simulink model "iot_casestudy_1_16"  (R2023a)
settings: Solver=VariableStepAuto  StartTime=0.0  StopTime=3.0  RelTol=1e-3
undefined symbols (not defined in the file or in its folder): m, n
(part 1 of 2)
settings Model: PacingRate=0.089000  Creator=simon  LastModifiedBy=simon
settings DataIOCC: SignalLogging=off
settings OptimizationCC: AccelVerboseBuild=on

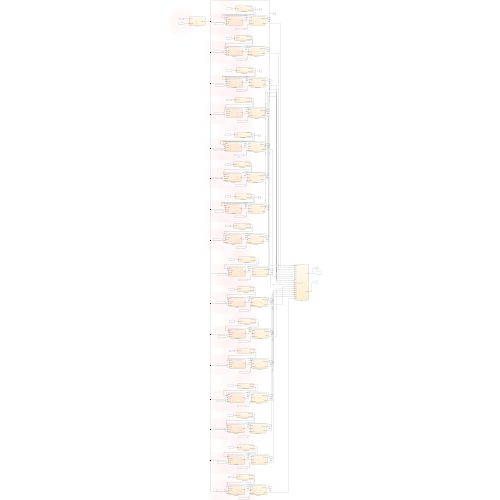
[thumbnail: Simulink's stored preview of the top-level diagram]
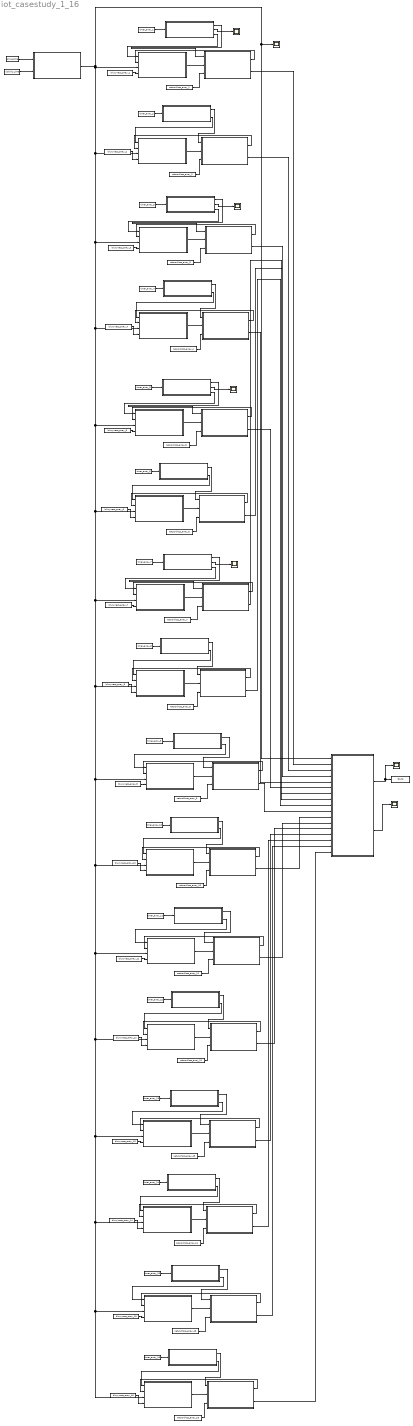
== system iot_casestudy_1_16 ==
  CameraControl : Stateflow chart  TreatAsAtomicUnit=on
      settings: PortSchema="{\"entries\":[{\"content\":{\"sides\":[{\"content\":{\"connectorIds\":[\"In3\",\"In1\",\"In2\"]},\"type\":\"ConnectorPlacement.EquallySpacedRectSide\",\"uuid\":\"ab620818-a51b-4a3c-9b00-600c4a6c30a0\"},{\"content\":{\"connectorIds\":[\"Out1\",\"Out2\"],\"side\":\"RIGHT\"},\"type\":\"ConnectorPlacement.EquallySpacedRectSide\",\"uuid\":\"fd7d4612-1aa1-44dc-acf4-0ffdcf3f06ab\"},{\"content\":{\"side\":\"TOP\"},\"type\":\"ConnectorPlacement.EquallySpacedRectSide\",\"uuid\":\"b173ad78-f658-4e97-9d6b-ed1d410de5f1\"}]},\"type\":\"ConnectorPlacement.EquallySpacedConnector\",\"uuid\":\"5700aeec-8725-4d1d-b13d-0f47828af58c\"}],\"packageUris\":[\"http://schema.mathworks.com/mf0/Connector/R2020b\"],\"version\":\"1.0\"}"
  CameraControl1 : Stateflow chart  TreatAsAtomicUnit=on
      settings: PortSchema="{\"entries\":[{\"content\":{\"sides\":[{\"content\":{\"connectorIds\":[\"In3\",\"In1\",\"In2\"]},\"type\":\"ConnectorPlacement.EquallySpacedRectSide\",\"uuid\":\"ab620818-a51b-4a3c-9b00-600c4a6c30a0\"},{\"content\":{\"connectorIds\":[\"Out1\",\"Out2\"],\"side\":\"RIGHT\"},\"type\":\"ConnectorPlacement.EquallySpacedRectSide\",\"uuid\":\"fd7d4612-1aa1-44dc-acf4-0ffdcf3f06ab\"},{\"content\":{\"side\":\"TOP\"},\"type\":\"ConnectorPlacement.EquallySpacedRectSide\",\"uuid\":\"b173ad78-f658-4e97-9d6b-ed1d410de5f1\"}]},\"type\":\"ConnectorPlacement.EquallySpacedConnector\",\"uuid\":\"5700aeec-8725-4d1d-b13d-0f47828af58c\"}],\"packageUris\":[\"http://schema.mathworks.com/mf0/Connector/R2020b\"],\"version\":\"1.0\"}"
  CameraControl10 : Stateflow chart  TreatAsAtomicUnit=on
      settings: PortSchema="{\"entries\":[{\"content\":{\"sides\":[{\"content\":{\"connectorIds\":[\"In3\",\"In1\",\"In2\"]},\"type\":\"ConnectorPlacement.EquallySpacedRectSide\",\"uuid\":\"ab620818-a51b-4a3c-9b00-600c4a6c30a0\"},{\"content\":{\"connectorIds\":[\"Out1\",\"Out2\"],\"side\":\"RIGHT\"},\"type\":\"ConnectorPlacement.EquallySpacedRectSide\",\"uuid\":\"fd7d4612-1aa1-44dc-acf4-0ffdcf3f06ab\"},{\"content\":{\"side\":\"TOP\"},\"type\":\"ConnectorPlacement.EquallySpacedRectSide\",\"uuid\":\"b173ad78-f658-4e97-9d6b-ed1d410de5f1\"}]},\"type\":\"ConnectorPlacement.EquallySpacedConnector\",\"uuid\":\"5700aeec-8725-4d1d-b13d-0f47828af58c\"}],\"packageUris\":[\"http://schema.mathworks.com/mf0/Connector/R2020b\"],\"version\":\"1.0\"}"
  CameraControl11 : Stateflow chart  TreatAsAtomicUnit=on
      settings: PortSchema="{\"entries\":[{\"content\":{\"sides\":[{\"content\":{\"connectorIds\":[\"In3\",\"In1\",\"In2\"]},\"type\":\"ConnectorPlacement.EquallySpacedRectSide\",\"uuid\":\"ab620818-a51b-4a3c-9b00-600c4a6c30a0\"},{\"content\":{\"connectorIds\":[\"Out1\",\"Out2\"],\"side\":\"RIGHT\"},\"type\":\"ConnectorPlacement.EquallySpacedRectSide\",\"uuid\":\"fd7d4612-1aa1-44dc-acf4-0ffdcf3f06ab\"},{\"content\":{\"side\":\"TOP\"},\"type\":\"ConnectorPlacement.EquallySpacedRectSide\",\"uuid\":\"b173ad78-f658-4e97-9d6b-ed1d410de5f1\"}]},\"type\":\"ConnectorPlacement.EquallySpacedConnector\",\"uuid\":\"5700aeec-8725-4d1d-b13d-0f47828af58c\"}],\"packageUris\":[\"http://schema.mathworks.com/mf0/Connector/R2020b\"],\"version\":\"1.0\"}"
  CameraControl12 : Stateflow chart  TreatAsAtomicUnit=on
      settings: PortSchema="{\"entries\":[{\"content\":{\"sides\":[{\"content\":{\"connectorIds\":[\"In3\",\"In1\",\"In2\"]},\"type\":\"ConnectorPlacement.EquallySpacedRectSide\",\"uuid\":\"ab620818-a51b-4a3c-9b00-600c4a6c30a0\"},{\"content\":{\"connectorIds\":[\"Out1\",\"Out2\"],\"side\":\"RIGHT\"},\"type\":\"ConnectorPlacement.EquallySpacedRectSide\",\"uuid\":\"fd7d4612-1aa1-44dc-acf4-0ffdcf3f06ab\"},{\"content\":{\"side\":\"TOP\"},\"type\":\"ConnectorPlacement.EquallySpacedRectSide\",\"uuid\":\"b173ad78-f658-4e97-9d6b-ed1d410de5f1\"}]},\"type\":\"ConnectorPlacement.EquallySpacedConnector\",\"uuid\":\"5700aeec-8725-4d1d-b13d-0f47828af58c\"}],\"packageUris\":[\"http://schema.mathworks.com/mf0/Connector/R2020b\"],\"version\":\"1.0\"}"
  CameraControl13 : Stateflow chart  TreatAsAtomicUnit=on
      settings: PortSchema="{\"entries\":[{\"content\":{\"sides\":[{\"content\":{\"connectorIds\":[\"In3\",\"In1\",\"In2\"]},\"type\":\"ConnectorPlacement.EquallySpacedRectSide\",\"uuid\":\"ab620818-a51b-4a3c-9b00-600c4a6c30a0\"},{\"content\":{\"connectorIds\":[\"Out1\",\"Out2\"],\"side\":\"RIGHT\"},\"type\":\"ConnectorPlacement.EquallySpacedRectSide\",\"uuid\":\"fd7d4612-1aa1-44dc-acf4-0ffdcf3f06ab\"},{\"content\":{\"side\":\"TOP\"},\"type\":\"ConnectorPlacement.EquallySpacedRectSide\",\"uuid\":\"b173ad78-f658-4e97-9d6b-ed1d410de5f1\"}]},\"type\":\"ConnectorPlacement.EquallySpacedConnector\",\"uuid\":\"5700aeec-8725-4d1d-b13d-0f47828af58c\"}],\"packageUris\":[\"http://schema.mathworks.com/mf0/Connector/R2020b\"],\"version\":\"1.0\"}"
  CameraControl14 : Stateflow chart  TreatAsAtomicUnit=on
      settings: PortSchema="{\"entries\":[{\"content\":{\"sides\":[{\"content\":{\"connectorIds\":[\"In3\",\"In1\",\"In2\"]},\"type\":\"ConnectorPlacement.EquallySpacedRectSide\",\"uuid\":\"ab620818-a51b-4a3c-9b00-600c4a6c30a0\"},{\"content\":{\"connectorIds\":[\"Out1\",\"Out2\"],\"side\":\"RIGHT\"},\"type\":\"ConnectorPlacement.EquallySpacedRectSide\",\"uuid\":\"fd7d4612-1aa1-44dc-acf4-0ffdcf3f06ab\"},{\"content\":{\"side\":\"TOP\"},\"type\":\"ConnectorPlacement.EquallySpacedRectSide\",\"uuid\":\"b173ad78-f658-4e97-9d6b-ed1d410de5f1\"}]},\"type\":\"ConnectorPlacement.EquallySpacedConnector\",\"uuid\":\"5700aeec-8725-4d1d-b13d-0f47828af58c\"}],\"packageUris\":[\"http://schema.mathworks.com/mf0/Connector/R2020b\"],\"version\":\"1.0\"}"
  CameraControl15 : Stateflow chart  TreatAsAtomicUnit=on
      settings: PortSchema="{\"entries\":[{\"content\":{\"sides\":[{\"content\":{\"connectorIds\":[\"In3\",\"In1\",\"In2\"]},\"type\":\"ConnectorPlacement.EquallySpacedRectSide\",\"uuid\":\"ab620818-a51b-4a3c-9b00-600c4a6c30a0\"},{\"content\":{\"connectorIds\":[\"Out1\",\"Out2\"],\"side\":\"RIGHT\"},\"type\":\"ConnectorPlacement.EquallySpacedRectSide\",\"uuid\":\"fd7d4612-1aa1-44dc-acf4-0ffdcf3f06ab\"},{\"content\":{\"side\":\"TOP\"},\"type\":\"ConnectorPlacement.EquallySpacedRectSide\",\"uuid\":\"b173ad78-f658-4e97-9d6b-ed1d410de5f1\"}]},\"type\":\"ConnectorPlacement.EquallySpacedConnector\",\"uuid\":\"5700aeec-8725-4d1d-b13d-0f47828af58c\"}],\"packageUris\":[\"http://schema.mathworks.com/mf0/Connector/R2020b\"],\"version\":\"1.0\"}"
  CameraControl2 : Stateflow chart  TreatAsAtomicUnit=on
      settings: PortSchema="{\"entries\":[{\"content\":{\"sides\":[{\"content\":{\"connectorIds\":[\"In3\",\"In1\",\"In2\"]},\"type\":\"ConnectorPlacement.EquallySpacedRectSide\",\"uuid\":\"ab620818-a51b-4a3c-9b00-600c4a6c30a0\"},{\"content\":{\"connectorIds\":[\"Out1\",\"Out2\"],\"side\":\"RIGHT\"},\"type\":\"ConnectorPlacement.EquallySpacedRectSide\",\"uuid\":\"fd7d4612-1aa1-44dc-acf4-0ffdcf3f06ab\"},{\"content\":{\"side\":\"TOP\"},\"type\":\"ConnectorPlacement.EquallySpacedRectSide\",\"uuid\":\"b173ad78-f658-4e97-9d6b-ed1d410de5f1\"}]},\"type\":\"ConnectorPlacement.EquallySpacedConnector\",\"uuid\":\"5700aeec-8725-4d1d-b13d-0f47828af58c\"}],\"packageUris\":[\"http://schema.mathworks.com/mf0/Connector/R2020b\"],\"version\":\"1.0\"}"
  CameraControl3 : Stateflow chart  TreatAsAtomicUnit=on
      settings: PortSchema="{\"entries\":[{\"content\":{\"sides\":[{\"content\":{\"connectorIds\":[\"In3\",\"In1\",\"In2\"]},\"type\":\"ConnectorPlacement.EquallySpacedRectSide\",\"uuid\":\"ab620818-a51b-4a3c-9b00-600c4a6c30a0\"},{\"content\":{\"connectorIds\":[\"Out1\",\"Out2\"],\"side\":\"RIGHT\"},\"type\":\"ConnectorPlacement.EquallySpacedRectSide\",\"uuid\":\"fd7d4612-1aa1-44dc-acf4-0ffdcf3f06ab\"},{\"content\":{\"side\":\"TOP\"},\"type\":\"ConnectorPlacement.EquallySpacedRectSide\",\"uuid\":\"b173ad78-f658-4e97-9d6b-ed1d410de5f1\"}]},\"type\":\"ConnectorPlacement.EquallySpacedConnector\",\"uuid\":\"5700aeec-8725-4d1d-b13d-0f47828af58c\"}],\"packageUris\":[\"http://schema.mathworks.com/mf0/Connector/R2020b\"],\"version\":\"1.0\"}"
  CameraControl4 : Stateflow chart  TreatAsAtomicUnit=on
      settings: PortSchema="{\"entries\":[{\"content\":{\"sides\":[{\"content\":{\"connectorIds\":[\"In3\",\"In1\",\"In2\"]},\"type\":\"ConnectorPlacement.EquallySpacedRectSide\",\"uuid\":\"ab620818-a51b-4a3c-9b00-600c4a6c30a0\"},{\"content\":{\"connectorIds\":[\"Out1\",\"Out2\"],\"side\":\"RIGHT\"},\"type\":\"ConnectorPlacement.EquallySpacedRectSide\",\"uuid\":\"fd7d4612-1aa1-44dc-acf4-0ffdcf3f06ab\"},{\"content\":{\"side\":\"TOP\"},\"type\":\"ConnectorPlacement.EquallySpacedRectSide\",\"uuid\":\"b173ad78-f658-4e97-9d6b-ed1d410de5f1\"}]},\"type\":\"ConnectorPlacement.EquallySpacedConnector\",\"uuid\":\"5700aeec-8725-4d1d-b13d-0f47828af58c\"}],\"packageUris\":[\"http://schema.mathworks.com/mf0/Connector/R2020b\"],\"version\":\"1.0\"}"
  CameraControl5 : Stateflow chart  TreatAsAtomicUnit=on
      settings: PortSchema="{\"entries\":[{\"content\":{\"sides\":[{\"content\":{\"connectorIds\":[\"In3\",\"In1\",\"In2\"]},\"type\":\"ConnectorPlacement.EquallySpacedRectSide\",\"uuid\":\"ab620818-a51b-4a3c-9b00-600c4a6c30a0\"},{\"content\":{\"connectorIds\":[\"Out1\",\"Out2\"],\"side\":\"RIGHT\"},\"type\":\"ConnectorPlacement.EquallySpacedRectSide\",\"uuid\":\"fd7d4612-1aa1-44dc-acf4-0ffdcf3f06ab\"},{\"content\":{\"side\":\"TOP\"},\"type\":\"ConnectorPlacement.EquallySpacedRectSide\",\"uuid\":\"b173ad78-f658-4e97-9d6b-ed1d410de5f1\"}]},\"type\":\"ConnectorPlacement.EquallySpacedConnector\",\"uuid\":\"5700aeec-8725-4d1d-b13d-0f47828af58c\"}],\"packageUris\":[\"http://schema.mathworks.com/mf0/Connector/R2020b\"],\"version\":\"1.0\"}"
  CameraControl6 : Stateflow chart  TreatAsAtomicUnit=on
      settings: PortSchema="{\"entries\":[{\"content\":{\"sides\":[{\"content\":{\"connectorIds\":[\"In3\",\"In1\",\"In2\"]},\"type\":\"ConnectorPlacement.EquallySpacedRectSide\",\"uuid\":\"ab620818-a51b-4a3c-9b00-600c4a6c30a0\"},{\"content\":{\"connectorIds\":[\"Out1\",\"Out2\"],\"side\":\"RIGHT\"},\"type\":\"ConnectorPlacement.EquallySpacedRectSide\",\"uuid\":\"fd7d4612-1aa1-44dc-acf4-0ffdcf3f06ab\"},{\"content\":{\"side\":\"TOP\"},\"type\":\"ConnectorPlacement.EquallySpacedRectSide\",\"uuid\":\"b173ad78-f658-4e97-9d6b-ed1d410de5f1\"}]},\"type\":\"ConnectorPlacement.EquallySpacedConnector\",\"uuid\":\"5700aeec-8725-4d1d-b13d-0f47828af58c\"}],\"packageUris\":[\"http://schema.mathworks.com/mf0/Connector/R2020b\"],\"version\":\"1.0\"}"
  CameraControl7 : Stateflow chart  TreatAsAtomicUnit=on
      settings: PortSchema="{\"entries\":[{\"content\":{\"sides\":[{\"content\":{\"connectorIds\":[\"In3\",\"In1\",\"In2\"]},\"type\":\"ConnectorPlacement.EquallySpacedRectSide\",\"uuid\":\"ab620818-a51b-4a3c-9b00-600c4a6c30a0\"},{\"content\":{\"connectorIds\":[\"Out1\",\"Out2\"],\"side\":\"RIGHT\"},\"type\":\"ConnectorPlacement.EquallySpacedRectSide\",\"uuid\":\"fd7d4612-1aa1-44dc-acf4-0ffdcf3f06ab\"},{\"content\":{\"side\":\"TOP\"},\"type\":\"ConnectorPlacement.EquallySpacedRectSide\",\"uuid\":\"b173ad78-f658-4e97-9d6b-ed1d410de5f1\"}]},\"type\":\"ConnectorPlacement.EquallySpacedConnector\",\"uuid\":\"5700aeec-8725-4d1d-b13d-0f47828af58c\"}],\"packageUris\":[\"http://schema.mathworks.com/mf0/Connector/R2020b\"],\"version\":\"1.0\"}"
  CameraControl8 : Stateflow chart  TreatAsAtomicUnit=on
      settings: PortSchema="{\"entries\":[{\"content\":{\"sides\":[{\"content\":{\"connectorIds\":[\"In3\",\"In1\",\"In2\"]},\"type\":\"ConnectorPlacement.EquallySpacedRectSide\",\"uuid\":\"ab620818-a51b-4a3c-9b00-600c4a6c30a0\"},{\"content\":{\"connectorIds\":[\"Out1\",\"Out2\"],\"side\":\"RIGHT\"},\"type\":\"ConnectorPlacement.EquallySpacedRectSide\",\"uuid\":\"fd7d4612-1aa1-44dc-acf4-0ffdcf3f06ab\"},{\"content\":{\"side\":\"TOP\"},\"type\":\"ConnectorPlacement.EquallySpacedRectSide\",\"uuid\":\"b173ad78-f658-4e97-9d6b-ed1d410de5f1\"}]},\"type\":\"ConnectorPlacement.EquallySpacedConnector\",\"uuid\":\"5700aeec-8725-4d1d-b13d-0f47828af58c\"}],\"packageUris\":[\"http://schema.mathworks.com/mf0/Connector/R2020b\"],\"version\":\"1.0\"}"
  CameraControl9 : Stateflow chart  TreatAsAtomicUnit=on
      settings: PortSchema="{\"entries\":[{\"content\":{\"sides\":[{\"content\":{\"connectorIds\":[\"In3\",\"In1\",\"In2\"]},\"type\":\"ConnectorPlacement.EquallySpacedRectSide\",\"uuid\":\"ab620818-a51b-4a3c-9b00-600c4a6c30a0\"},{\"content\":{\"connectorIds\":[\"Out1\",\"Out2\"],\"side\":\"RIGHT\"},\"type\":\"ConnectorPlacement.EquallySpacedRectSide\",\"uuid\":\"fd7d4612-1aa1-44dc-acf4-0ffdcf3f06ab\"},{\"content\":{\"side\":\"TOP\"},\"type\":\"ConnectorPlacement.EquallySpacedRectSide\",\"uuid\":\"b173ad78-f658-4e97-9d6b-ed1d410de5f1\"}]},\"type\":\"ConnectorPlacement.EquallySpacedConnector\",\"uuid\":\"5700aeec-8725-4d1d-b13d-0f47828af58c\"}],\"packageUris\":[\"http://schema.mathworks.com/mf0/Connector/R2020b\"],\"version\":\"1.0\"}"
  CameraDriver : Stateflow chart  TreatAsAtomicUnit=on
      settings: PortSchema="{\"entries\":[{\"content\":{\"sides\":[{\"content\":{\"connectorIds\":[\"In4\",\"In1\",\"In2\",\"In3\"]},\"type\":\"ConnectorPlacement.EquallySpacedRectSide\",\"uuid\":\"49bdffc0-8e15-4462-b991-b36534669558\"},{\"content\":{\"connectorIds\":[\"Out1\"],\"side\":\"RIGHT\"},\"type\":\"ConnectorPlacement.EquallySpacedRectSide\",\"uuid\":\"379950e5-a8e3-41fb-8f45-c3d731cfbd8a\"},{\"content\":{\"side\":\"TOP\"},\"type\":\"ConnectorPlacement.EquallySpacedRectSide\",\"uuid\":\"38309075-1b62-4fbc-9171-ddac584f70df\"}]},\"type\":\"ConnectorPlacement.EquallySpacedConnector\",\"uuid\":\"335a78c7-f6bb-4aff-a350-269f860e2554\"}],\"packageUris\":[\"http://schema.mathworks.com/mf0/Connector/R2020b\"],\"version\":\"1.0\"}"
  CameraDriver1 : Stateflow chart  TreatAsAtomicUnit=on
      settings: PortSchema="{\"entries\":[{\"content\":{\"sides\":[{\"content\":{\"connectorIds\":[\"In4\",\"In1\",\"In2\",\"In3\"]},\"type\":\"ConnectorPlacement.EquallySpacedRectSide\",\"uuid\":\"49bdffc0-8e15-4462-b991-b36534669558\"},{\"content\":{\"connectorIds\":[\"Out1\"],\"side\":\"RIGHT\"},\"type\":\"ConnectorPlacement.EquallySpacedRectSide\",\"uuid\":\"379950e5-a8e3-41fb-8f45-c3d731cfbd8a\"},{\"content\":{\"side\":\"TOP\"},\"type\":\"ConnectorPlacement.EquallySpacedRectSide\",\"uuid\":\"38309075-1b62-4fbc-9171-ddac584f70df\"}]},\"type\":\"ConnectorPlacement.EquallySpacedConnector\",\"uuid\":\"335a78c7-f6bb-4aff-a350-269f860e2554\"}],\"packageUris\":[\"http://schema.mathworks.com/mf0/Connector/R2020b\"],\"version\":\"1.0\"}"
  CameraDriver10 : Stateflow chart  TreatAsAtomicUnit=on
      settings: PortSchema="{\"entries\":[{\"content\":{\"sides\":[{\"content\":{\"connectorIds\":[\"In4\",\"In1\",\"In2\",\"In3\"]},\"type\":\"ConnectorPlacement.EquallySpacedRectSide\",\"uuid\":\"49bdffc0-8e15-4462-b991-b36534669558\"},{\"content\":{\"connectorIds\":[\"Out1\"],\"side\":\"RIGHT\"},\"type\":\"ConnectorPlacement.EquallySpacedRectSide\",\"uuid\":\"379950e5-a8e3-41fb-8f45-c3d731cfbd8a\"},{\"content\":{\"side\":\"TOP\"},\"type\":\"ConnectorPlacement.EquallySpacedRectSide\",\"uuid\":\"38309075-1b62-4fbc-9171-ddac584f70df\"}]},\"type\":\"ConnectorPlacement.EquallySpacedConnector\",\"uuid\":\"335a78c7-f6bb-4aff-a350-269f860e2554\"}],\"packageUris\":[\"http://schema.mathworks.com/mf0/Connector/R2020b\"],\"version\":\"1.0\"}"
  CameraDriver11 : Stateflow chart  TreatAsAtomicUnit=on
      settings: PortSchema="{\"entries\":[{\"content\":{\"sides\":[{\"content\":{\"connectorIds\":[\"In4\",\"In1\",\"In2\",\"In3\"]},\"type\":\"ConnectorPlacement.EquallySpacedRectSide\",\"uuid\":\"49bdffc0-8e15-4462-b991-b36534669558\"},{\"content\":{\"connectorIds\":[\"Out1\"],\"side\":\"RIGHT\"},\"type\":\"ConnectorPlacement.EquallySpacedRectSide\",\"uuid\":\"379950e5-a8e3-41fb-8f45-c3d731cfbd8a\"},{\"content\":{\"side\":\"TOP\"},\"type\":\"ConnectorPlacement.EquallySpacedRectSide\",\"uuid\":\"38309075-1b62-4fbc-9171-ddac584f70df\"}]},\"type\":\"ConnectorPlacement.EquallySpacedConnector\",\"uuid\":\"335a78c7-f6bb-4aff-a350-269f860e2554\"}],\"packageUris\":[\"http://schema.mathworks.com/mf0/Connector/R2020b\"],\"version\":\"1.0\"}"
  CameraDriver12 : Stateflow chart  TreatAsAtomicUnit=on
      settings: PortSchema="{\"entries\":[{\"content\":{\"sides\":[{\"content\":{\"connectorIds\":[\"In4\",\"In1\",\"In2\",\"In3\"]},\"type\":\"ConnectorPlacement.EquallySpacedRectSide\",\"uuid\":\"49bdffc0-8e15-4462-b991-b36534669558\"},{\"content\":{\"connectorIds\":[\"Out1\"],\"side\":\"RIGHT\"},\"type\":\"ConnectorPlacement.EquallySpacedRectSide\",\"uuid\":\"379950e5-a8e3-41fb-8f45-c3d731cfbd8a\"},{\"content\":{\"side\":\"TOP\"},\"type\":\"ConnectorPlacement.EquallySpacedRectSide\",\"uuid\":\"38309075-1b62-4fbc-9171-ddac584f70df\"}]},\"type\":\"ConnectorPlacement.EquallySpacedConnector\",\"uuid\":\"335a78c7-f6bb-4aff-a350-269f860e2554\"}],\"packageUris\":[\"http://schema.mathworks.com/mf0/Connector/R2020b\"],\"version\":\"1.0\"}"
  CameraDriver13 : Stateflow chart  TreatAsAtomicUnit=on
      settings: PortSchema="{\"entries\":[{\"content\":{\"sides\":[{\"content\":{\"connectorIds\":[\"In4\",\"In1\",\"In2\",\"In3\"]},\"type\":\"ConnectorPlacement.EquallySpacedRectSide\",\"uuid\":\"49bdffc0-8e15-4462-b991-b36534669558\"},{\"content\":{\"connectorIds\":[\"Out1\"],\"side\":\"RIGHT\"},\"type\":\"ConnectorPlacement.EquallySpacedRectSide\",\"uuid\":\"379950e5-a8e3-41fb-8f45-c3d731cfbd8a\"},{\"content\":{\"side\":\"TOP\"},\"type\":\"ConnectorPlacement.EquallySpacedRectSide\",\"uuid\":\"38309075-1b62-4fbc-9171-ddac584f70df\"}]},\"type\":\"ConnectorPlacement.EquallySpacedConnector\",\"uuid\":\"335a78c7-f6bb-4aff-a350-269f860e2554\"}],\"packageUris\":[\"http://schema.mathworks.com/mf0/Connector/R2020b\"],\"version\":\"1.0\"}"
  CameraDriver14 : Stateflow chart  TreatAsAtomicUnit=on
      settings: PortSchema="{\"entries\":[{\"content\":{\"sides\":[{\"content\":{\"connectorIds\":[\"In4\",\"In1\",\"In2\",\"In3\"]},\"type\":\"ConnectorPlacement.EquallySpacedRectSide\",\"uuid\":\"49bdffc0-8e15-4462-b991-b36534669558\"},{\"content\":{\"connectorIds\":[\"Out1\"],\"side\":\"RIGHT\"},\"type\":\"ConnectorPlacement.EquallySpacedRectSide\",\"uuid\":\"379950e5-a8e3-41fb-8f45-c3d731cfbd8a\"},{\"content\":{\"side\":\"TOP\"},\"type\":\"ConnectorPlacement.EquallySpacedRectSide\",\"uuid\":\"38309075-1b62-4fbc-9171-ddac584f70df\"}]},\"type\":\"ConnectorPlacement.EquallySpacedConnector\",\"uuid\":\"335a78c7-f6bb-4aff-a350-269f860e2554\"}],\"packageUris\":[\"http://schema.mathworks.com/mf0/Connector/R2020b\"],\"version\":\"1.0\"}"
  CameraDriver15 : Stateflow chart  TreatAsAtomicUnit=on
      settings: PortSchema="{\"entries\":[{\"content\":{\"sides\":[{\"content\":{\"connectorIds\":[\"In4\",\"In1\",\"In2\",\"In3\"]},\"type\":\"ConnectorPlacement.EquallySpacedRectSide\",\"uuid\":\"49bdffc0-8e15-4462-b991-b36534669558\"},{\"content\":{\"connectorIds\":[\"Out1\"],\"side\":\"RIGHT\"},\"type\":\"ConnectorPlacement.EquallySpacedRectSide\",\"uuid\":\"379950e5-a8e3-41fb-8f45-c3d731cfbd8a\"},{\"content\":{\"side\":\"TOP\"},\"type\":\"ConnectorPlacement.EquallySpacedRectSide\",\"uuid\":\"38309075-1b62-4fbc-9171-ddac584f70df\"}]},\"type\":\"ConnectorPlacement.EquallySpacedConnector\",\"uuid\":\"335a78c7-f6bb-4aff-a350-269f860e2554\"}],\"packageUris\":[\"http://schema.mathworks.com/mf0/Connector/R2020b\"],\"version\":\"1.0\"}"
  CameraDriver2 : Stateflow chart  TreatAsAtomicUnit=on
      settings: PortSchema="{\"entries\":[{\"content\":{\"sides\":[{\"content\":{\"connectorIds\":[\"In4\",\"In1\",\"In2\",\"In3\"]},\"type\":\"ConnectorPlacement.EquallySpacedRectSide\",\"uuid\":\"49bdffc0-8e15-4462-b991-b36534669558\"},{\"content\":{\"connectorIds\":[\"Out1\"],\"side\":\"RIGHT\"},\"type\":\"ConnectorPlacement.EquallySpacedRectSide\",\"uuid\":\"379950e5-a8e3-41fb-8f45-c3d731cfbd8a\"},{\"content\":{\"side\":\"TOP\"},\"type\":\"ConnectorPlacement.EquallySpacedRectSide\",\"uuid\":\"38309075-1b62-4fbc-9171-ddac584f70df\"}]},\"type\":\"ConnectorPlacement.EquallySpacedConnector\",\"uuid\":\"335a78c7-f6bb-4aff-a350-269f860e2554\"}],\"packageUris\":[\"http://schema.mathworks.com/mf0/Connector/R2020b\"],\"version\":\"1.0\"}"
  CameraDriver3 : Stateflow chart  TreatAsAtomicUnit=on
      settings: PortSchema="{\"entries\":[{\"content\":{\"sides\":[{\"content\":{\"connectorIds\":[\"In4\",\"In1\",\"In2\",\"In3\"]},\"type\":\"ConnectorPlacement.EquallySpacedRectSide\",\"uuid\":\"49bdffc0-8e15-4462-b991-b36534669558\"},{\"content\":{\"connectorIds\":[\"Out1\"],\"side\":\"RIGHT\"},\"type\":\"ConnectorPlacement.EquallySpacedRectSide\",\"uuid\":\"379950e5-a8e3-41fb-8f45-c3d731cfbd8a\"},{\"content\":{\"side\":\"TOP\"},\"type\":\"ConnectorPlacement.EquallySpacedRectSide\",\"uuid\":\"38309075-1b62-4fbc-9171-ddac584f70df\"}]},\"type\":\"ConnectorPlacement.EquallySpacedConnector\",\"uuid\":\"335a78c7-f6bb-4aff-a350-269f860e2554\"}],\"packageUris\":[\"http://schema.mathworks.com/mf0/Connector/R2020b\"],\"version\":\"1.0\"}"
  CameraDriver4 : Stateflow chart  TreatAsAtomicUnit=on
      settings: PortSchema="{\"entries\":[{\"content\":{\"sides\":[{\"content\":{\"connectorIds\":[\"In4\",\"In1\",\"In2\",\"In3\"]},\"type\":\"ConnectorPlacement.EquallySpacedRectSide\",\"uuid\":\"49bdffc0-8e15-4462-b991-b36534669558\"},{\"content\":{\"connectorIds\":[\"Out1\"],\"side\":\"RIGHT\"},\"type\":\"ConnectorPlacement.EquallySpacedRectSide\",\"uuid\":\"379950e5-a8e3-41fb-8f45-c3d731cfbd8a\"},{\"content\":{\"side\":\"TOP\"},\"type\":\"ConnectorPlacement.EquallySpacedRectSide\",\"uuid\":\"38309075-1b62-4fbc-9171-ddac584f70df\"}]},\"type\":\"ConnectorPlacement.EquallySpacedConnector\",\"uuid\":\"335a78c7-f6bb-4aff-a350-269f860e2554\"}],\"packageUris\":[\"http://schema.mathworks.com/mf0/Connector/R2020b\"],\"version\":\"1.0\"}"
  CameraDriver5 : Stateflow chart  TreatAsAtomicUnit=on
      settings: PortSchema="{\"entries\":[{\"content\":{\"sides\":[{\"content\":{\"connectorIds\":[\"In4\",\"In1\",\"In2\",\"In3\"]},\"type\":\"ConnectorPlacement.EquallySpacedRectSide\",\"uuid\":\"49bdffc0-8e15-4462-b991-b36534669558\"},{\"content\":{\"connectorIds\":[\"Out1\"],\"side\":\"RIGHT\"},\"type\":\"ConnectorPlacement.EquallySpacedRectSide\",\"uuid\":\"379950e5-a8e3-41fb-8f45-c3d731cfbd8a\"},{\"content\":{\"side\":\"TOP\"},\"type\":\"ConnectorPlacement.EquallySpacedRectSide\",\"uuid\":\"38309075-1b62-4fbc-9171-ddac584f70df\"}]},\"type\":\"ConnectorPlacement.EquallySpacedConnector\",\"uuid\":\"335a78c7-f6bb-4aff-a350-269f860e2554\"}],\"packageUris\":[\"http://schema.mathworks.com/mf0/Connector/R2020b\"],\"version\":\"1.0\"}"
  CameraDriver6 : Stateflow chart  TreatAsAtomicUnit=on
      settings: PortSchema="{\"entries\":[{\"content\":{\"sides\":[{\"content\":{\"connectorIds\":[\"In4\",\"In1\",\"In2\",\"In3\"]},\"type\":\"ConnectorPlacement.EquallySpacedRectSide\",\"uuid\":\"49bdffc0-8e15-4462-b991-b36534669558\"},{\"content\":{\"connectorIds\":[\"Out1\"],\"side\":\"RIGHT\"},\"type\":\"ConnectorPlacement.EquallySpacedRectSide\",\"uuid\":\"379950e5-a8e3-41fb-8f45-c3d731cfbd8a\"},{\"content\":{\"side\":\"TOP\"},\"type\":\"ConnectorPlacement.EquallySpacedRectSide\",\"uuid\":\"38309075-1b62-4fbc-9171-ddac584f70df\"}]},\"type\":\"ConnectorPlacement.EquallySpacedConnector\",\"uuid\":\"335a78c7-f6bb-4aff-a350-269f860e2554\"}],\"packageUris\":[\"http://schema.mathworks.com/mf0/Connector/R2020b\"],\"version\":\"1.0\"}"
  CameraDriver7 : Stateflow chart  TreatAsAtomicUnit=on
      settings: PortSchema="{\"entries\":[{\"content\":{\"sides\":[{\"content\":{\"connectorIds\":[\"In4\",\"In1\",\"In2\",\"In3\"]},\"type\":\"ConnectorPlacement.EquallySpacedRectSide\",\"uuid\":\"49bdffc0-8e15-4462-b991-b36534669558\"},{\"content\":{\"connectorIds\":[\"Out1\"],\"side\":\"RIGHT\"},\"type\":\"ConnectorPlacement.EquallySpacedRectSide\",\"uuid\":\"379950e5-a8e3-41fb-8f45-c3d731cfbd8a\"},{\"content\":{\"side\":\"TOP\"},\"type\":\"ConnectorPlacement.EquallySpacedRectSide\",\"uuid\":\"38309075-1b62-4fbc-9171-ddac584f70df\"}]},\"type\":\"ConnectorPlacement.EquallySpacedConnector\",\"uuid\":\"335a78c7-f6bb-4aff-a350-269f860e2554\"}],\"packageUris\":[\"http://schema.mathworks.com/mf0/Connector/R2020b\"],\"version\":\"1.0\"}"
  CameraDriver8 : Stateflow chart  TreatAsAtomicUnit=on
      settings: PortSchema="{\"entries\":[{\"content\":{\"sides\":[{\"content\":{\"connectorIds\":[\"In4\",\"In1\",\"In2\",\"In3\"]},\"type\":\"ConnectorPlacement.EquallySpacedRectSide\",\"uuid\":\"49bdffc0-8e15-4462-b991-b36534669558\"},{\"content\":{\"connectorIds\":[\"Out1\"],\"side\":\"RIGHT\"},\"type\":\"ConnectorPlacement.EquallySpacedRectSide\",\"uuid\":\"379950e5-a8e3-41fb-8f45-c3d731cfbd8a\"},{\"content\":{\"side\":\"TOP\"},\"type\":\"ConnectorPlacement.EquallySpacedRectSide\",\"uuid\":\"38309075-1b62-4fbc-9171-ddac584f70df\"}]},\"type\":\"ConnectorPlacement.EquallySpacedConnector\",\"uuid\":\"335a78c7-f6bb-4aff-a350-269f860e2554\"}],\"packageUris\":[\"http://schema.mathworks.com/mf0/Connector/R2020b\"],\"version\":\"1.0\"}"
  CameraDriver9 : Stateflow chart  TreatAsAtomicUnit=on
      settings: PortSchema="{\"entries\":[{\"content\":{\"sides\":[{\"content\":{\"connectorIds\":[\"In4\",\"In1\",\"In2\",\"In3\"]},\"type\":\"ConnectorPlacement.EquallySpacedRectSide\",\"uuid\":\"49bdffc0-8e15-4462-b991-b36534669558\"},{\"content\":{\"connectorIds\":[\"Out1\"],\"side\":\"RIGHT\"},\"type\":\"ConnectorPlacement.EquallySpacedRectSide\",\"uuid\":\"379950e5-a8e3-41fb-8f45-c3d731cfbd8a\"},{\"content\":{\"side\":\"TOP\"},\"type\":\"ConnectorPlacement.EquallySpacedRectSide\",\"uuid\":\"38309075-1b62-4fbc-9171-ddac584f70df\"}]},\"type\":\"ConnectorPlacement.EquallySpacedConnector\",\"uuid\":\"335a78c7-f6bb-4aff-a350-269f860e2554\"}],\"packageUris\":[\"http://schema.mathworks.com/mf0/Connector/R2020b\"],\"version\":\"1.0\"}"
  CameraScheduler : Stateflow chart  TreatAsAtomicUnit=on
      settings: PortSchema="{\"entries\":[{\"content\":{\"sides\":[{\"content\":{\"connectorIds\":[\"In1\"]},\"type\":\"ConnectorPlacement.EquallySpacedRectSide\",\"uuid\":\"228150a7-62a2-46d0-a1ac-a8e868d835b5\"},{\"content\":{\"connectorIds\":[\"Out2\",\"Out3\",\"Out1\"],\"side\":\"RIGHT\"},\"type\":\"ConnectorPlacement.EquallySpacedRectSide\",\"uuid\":\"cb1c6840-c5bf-4913-92c2-1c054d368f87\"},{\"content\":{\"side\":\"TOP\"},\"type\":\"ConnectorPlacement.EquallySpacedRectSide\",\"uuid\":\"3633cd87-b3f9-48c9-80b7-73d7f17aa7ad\"}]},\"type\":\"ConnectorPlacement.EquallySpacedConnector\",\"uuid\":\"2553d532-cb7a-499b-b98c-b91f81677a07\"}],\"packageUris\":[\"http://schema.mathworks.com/mf0/Connector/R2020b\"],\"version\":\"1.0\"}"
  CameraScheduler1 : Stateflow chart  TreatAsAtomicUnit=on
      settings: PortSchema="{\"entries\":[{\"content\":{\"sides\":[{\"content\":{\"connectorIds\":[\"In1\"]},\"type\":\"ConnectorPlacement.EquallySpacedRectSide\",\"uuid\":\"335362b2-4c4f-40e6-baf0-d287f6971824\"},{\"content\":{\"connectorIds\":[\"Out2\",\"Out1\"],\"side\":\"RIGHT\"},\"type\":\"ConnectorPlacement.EquallySpacedRectSide\",\"uuid\":\"7ee54d08-aa3e-4d6f-8253-6f749626479a\"},{\"content\":{\"side\":\"TOP\"},\"type\":\"ConnectorPlacement.EquallySpacedRectSide\",\"uuid\":\"7bf47310-47f4-4483-b0d1-b8a087b66b77\"}]},\"type\":\"ConnectorPlacement.EquallySpacedConnector\",\"uuid\":\"fb61df21-9632-41f0-9cfa-ce5060944b6c\"}],\"packageUris\":[\"http://schema.mathworks.com/mf0/Connector/R2020b\"],\"version\":\"1.0\"}"
  CameraScheduler10 : Stateflow chart  TreatAsAtomicUnit=on
      settings: PortSchema="{\"entries\":[{\"content\":{\"sides\":[{\"content\":{\"connectorIds\":[\"In1\"]},\"type\":\"ConnectorPlacement.EquallySpacedRectSide\",\"uuid\":\"228150a7-62a2-46d0-a1ac-a8e868d835b5\"},{\"content\":{\"connectorIds\":[\"Out2\",\"Out1\"],\"side\":\"RIGHT\"},\"type\":\"ConnectorPlacement.EquallySpacedRectSide\",\"uuid\":\"cb1c6840-c5bf-4913-92c2-1c054d368f87\"},{\"content\":{\"side\":\"TOP\"},\"type\":\"ConnectorPlacement.EquallySpacedRectSide\",\"uuid\":\"3633cd87-b3f9-48c9-80b7-73d7f17aa7ad\"}]},\"type\":\"ConnectorPlacement.EquallySpacedConnector\",\"uuid\":\"2553d532-cb7a-499b-b98c-b91f81677a07\"}],\"packageUris\":[\"http://schema.mathworks.com/mf0/Connector/R2020b\"],\"version\":\"1.0\"}"
  CameraScheduler11 : Stateflow chart  TreatAsAtomicUnit=on
      settings: PortSchema="{\"entries\":[{\"content\":{\"sides\":[{\"content\":{\"connectorIds\":[\"In1\"]},\"type\":\"ConnectorPlacement.EquallySpacedRectSide\",\"uuid\":\"335362b2-4c4f-40e6-baf0-d287f6971824\"},{\"content\":{\"connectorIds\":[\"Out2\",\"Out1\"],\"side\":\"RIGHT\"},\"type\":\"ConnectorPlacement.EquallySpacedRectSide\",\"uuid\":\"7ee54d08-aa3e-4d6f-8253-6f749626479a\"},{\"content\":{\"side\":\"TOP\"},\"type\":\"ConnectorPlacement.EquallySpacedRectSide\",\"uuid\":\"7bf47310-47f4-4483-b0d1-b8a087b66b77\"}]},\"type\":\"ConnectorPlacement.EquallySpacedConnector\",\"uuid\":\"fb61df21-9632-41f0-9cfa-ce5060944b6c\"}],\"packageUris\":[\"http://schema.mathworks.com/mf0/Connector/R2020b\"],\"version\":\"1.0\"}"
  CameraScheduler12 : Stateflow chart  TreatAsAtomicUnit=on
      settings: PortSchema="{\"entries\":[{\"content\":{\"sides\":[{\"content\":{\"connectorIds\":[\"In1\"]},\"type\":\"ConnectorPlacement.EquallySpacedRectSide\",\"uuid\":\"228150a7-62a2-46d0-a1ac-a8e868d835b5\"},{\"content\":{\"connectorIds\":[\"Out2\",\"Out1\"],\"side\":\"RIGHT\"},\"type\":\"ConnectorPlacement.EquallySpacedRectSide\",\"uuid\":\"cb1c6840-c5bf-4913-92c2-1c054d368f87\"},{\"content\":{\"side\":\"TOP\"},\"type\":\"ConnectorPlacement.EquallySpacedRectSide\",\"uuid\":\"3633cd87-b3f9-48c9-80b7-73d7f17aa7ad\"}]},\"type\":\"ConnectorPlacement.EquallySpacedConnector\",\"uuid\":\"2553d532-cb7a-499b-b98c-b91f81677a07\"}],\"packageUris\":[\"http://schema.mathworks.com/mf0/Connector/R2020b\"],\"version\":\"1.0\"}"
  CameraScheduler13 : Stateflow chart  TreatAsAtomicUnit=on
      settings: PortSchema="{\"entries\":[{\"content\":{\"sides\":[{\"content\":{\"connectorIds\":[\"In1\"]},\"type\":\"ConnectorPlacement.EquallySpacedRectSide\",\"uuid\":\"335362b2-4c4f-40e6-baf0-d287f6971824\"},{\"content\":{\"connectorIds\":[\"Out2\",\"Out1\"],\"side\":\"RIGHT\"},\"type\":\"ConnectorPlacement.EquallySpacedRectSide\",\"uuid\":\"7ee54d08-aa3e-4d6f-8253-6f749626479a\"},{\"content\":{\"side\":\"TOP\"},\"type\":\"ConnectorPlacement.EquallySpacedRectSide\",\"uuid\":\"7bf47310-47f4-4483-b0d1-b8a087b66b77\"}]},\"type\":\"ConnectorPlacement.EquallySpacedConnector\",\"uuid\":\"fb61df21-9632-41f0-9cfa-ce5060944b6c\"}],\"packageUris\":[\"http://schema.mathworks.com/mf0/Connector/R2020b\"],\"version\":\"1.0\"}"
  CameraScheduler14 : Stateflow chart  TreatAsAtomicUnit=on
      settings: PortSchema="{\"entries\":[{\"content\":{\"sides\":[{\"content\":{\"connectorIds\":[\"In1\"]},\"type\":\"ConnectorPlacement.EquallySpacedRectSide\",\"uuid\":\"228150a7-62a2-46d0-a1ac-a8e868d835b5\"},{\"content\":{\"connectorIds\":[\"Out2\",\"Out1\"],\"side\":\"RIGHT\"},\"type\":\"ConnectorPlacement.EquallySpacedRectSide\",\"uuid\":\"cb1c6840-c5bf-4913-92c2-1c054d368f87\"},{\"content\":{\"side\":\"TOP\"},\"type\":\"ConnectorPlacement.EquallySpacedRectSide\",\"uuid\":\"3633cd87-b3f9-48c9-80b7-73d7f17aa7ad\"}]},\"type\":\"ConnectorPlacement.EquallySpacedConnector\",\"uuid\":\"2553d532-cb7a-499b-b98c-b91f81677a07\"}],\"packageUris\":[\"http://schema.mathworks.com/mf0/Connector/R2020b\"],\"version\":\"1.0\"}"
  CameraScheduler15 : Stateflow chart  TreatAsAtomicUnit=on
      settings: PortSchema="{\"entries\":[{\"content\":{\"sides\":[{\"content\":{\"connectorIds\":[\"In1\"]},\"type\":\"ConnectorPlacement.EquallySpacedRectSide\",\"uuid\":\"335362b2-4c4f-40e6-baf0-d287f6971824\"},{\"content\":{\"connectorIds\":[\"Out2\",\"Out1\"],\"side\":\"RIGHT\"},\"type\":\"ConnectorPlacement.EquallySpacedRectSide\",\"uuid\":\"7ee54d08-aa3e-4d6f-8253-6f749626479a\"},{\"content\":{\"side\":\"TOP\"},\"type\":\"ConnectorPlacement.EquallySpacedRectSide\",\"uuid\":\"7bf47310-47f4-4483-b0d1-b8a087b66b77\"}]},\"type\":\"ConnectorPlacement.EquallySpacedConnector\",\"uuid\":\"fb61df21-9632-41f0-9cfa-ce5060944b6c\"}],\"packageUris\":[\"http://schema.mathworks.com/mf0/Connector/R2020b\"],\"version\":\"1.0\"}"
  CameraScheduler2 : Stateflow chart  TreatAsAtomicUnit=on
      settings: PortSchema="{\"entries\":[{\"content\":{\"sides\":[{\"content\":{\"connectorIds\":[\"In1\"]},\"type\":\"ConnectorPlacement.EquallySpacedRectSide\",\"uuid\":\"228150a7-62a2-46d0-a1ac-a8e868d835b5\"},{\"content\":{\"connectorIds\":[\"Out2\",\"Out3\",\"Out1\"],\"side\":\"RIGHT\"},\"type\":\"ConnectorPlacement.EquallySpacedRectSide\",\"uuid\":\"cb1c6840-c5bf-4913-92c2-1c054d368f87\"},{\"content\":{\"side\":\"TOP\"},\"type\":\"ConnectorPlacement.EquallySpacedRectSide\",\"uuid\":\"3633cd87-b3f9-48c9-80b7-73d7f17aa7ad\"}]},\"type\":\"ConnectorPlacement.EquallySpacedConnector\",\"uuid\":\"2553d532-cb7a-499b-b98c-b91f81677a07\"}],\"packageUris\":[\"http://schema.mathworks.com/mf0/Connector/R2020b\"],\"version\":\"1.0\"}"
  CameraScheduler3 : Stateflow chart  TreatAsAtomicUnit=on
      settings: PortSchema="{\"entries\":[{\"content\":{\"sides\":[{\"content\":{\"connectorIds\":[\"In1\"]},\"type\":\"ConnectorPlacement.EquallySpacedRectSide\",\"uuid\":\"335362b2-4c4f-40e6-baf0-d287f6971824\"},{\"content\":{\"connectorIds\":[\"Out2\",\"Out1\"],\"side\":\"RIGHT\"},\"type\":\"ConnectorPlacement.EquallySpacedRectSide\",\"uuid\":\"7ee54d08-aa3e-4d6f-8253-6f749626479a\"},{\"content\":{\"side\":\"TOP\"},\"type\":\"ConnectorPlacement.EquallySpacedRectSide\",\"uuid\":\"7bf47310-47f4-4483-b0d1-b8a087b66b77\"}]},\"type\":\"ConnectorPlacement.EquallySpacedConnector\",\"uuid\":\"fb61df21-9632-41f0-9cfa-ce5060944b6c\"}],\"packageUris\":[\"http://schema.mathworks.com/mf0/Connector/R2020b\"],\"version\":\"1.0\"}"
  CameraScheduler4 : Stateflow chart  TreatAsAtomicUnit=on
      settings: PortSchema="{\"entries\":[{\"content\":{\"sides\":[{\"content\":{\"connectorIds\":[\"In1\"]},\"type\":\"ConnectorPlacement.EquallySpacedRectSide\",\"uuid\":\"228150a7-62a2-46d0-a1ac-a8e868d835b5\"},{\"content\":{\"connectorIds\":[\"Out2\",\"Out3\",\"Out1\"],\"side\":\"RIGHT\"},\"type\":\"ConnectorPlacement.EquallySpacedRectSide\",\"uuid\":\"cb1c6840-c5bf-4913-92c2-1c054d368f87\"},{\"content\":{\"side\":\"TOP\"},\"type\":\"ConnectorPlacement.EquallySpacedRectSide\",\"uuid\":\"3633cd87-b3f9-48c9-80b7-73d7f17aa7ad\"}]},\"type\":\"ConnectorPlacement.EquallySpacedConnector\",\"uuid\":\"2553d532-cb7a-499b-b98c-b91f81677a07\"}],\"packageUris\":[\"http://schema.mathworks.com/mf0/Connector/R2020b\"],\"version\":\"1.0\"}"
  CameraScheduler5 : Stateflow chart  TreatAsAtomicUnit=on
      settings: PortSchema="{\"entries\":[{\"content\":{\"sides\":[{\"content\":{\"connectorIds\":[\"In1\"]},\"type\":\"ConnectorPlacement.EquallySpacedRectSide\",\"uuid\":\"335362b2-4c4f-40e6-baf0-d287f6971824\"},{\"content\":{\"connectorIds\":[\"Out2\",\"Out1\"],\"side\":\"RIGHT\"},\"type\":\"ConnectorPlacement.EquallySpacedRectSide\",\"uuid\":\"7ee54d08-aa3e-4d6f-8253-6f749626479a\"},{\"content\":{\"side\":\"TOP\"},\"type\":\"ConnectorPlacement.EquallySpacedRectSide\",\"uuid\":\"7bf47310-47f4-4483-b0d1-b8a087b66b77\"}]},\"type\":\"ConnectorPlacement.EquallySpacedConnector\",\"uuid\":\"fb61df21-9632-41f0-9cfa-ce5060944b6c\"}],\"packageUris\":[\"http://schema.mathworks.com/mf0/Connector/R2020b\"],\"version\":\"1.0\"}"
  CameraScheduler6 : Stateflow chart  TreatAsAtomicUnit=on
      settings: PortSchema="{\"entries\":[{\"content\":{\"sides\":[{\"content\":{\"connectorIds\":[\"In1\"]},\"type\":\"ConnectorPlacement.EquallySpacedRectSide\",\"uuid\":\"228150a7-62a2-46d0-a1ac-a8e868d835b5\"},{\"content\":{\"connectorIds\":[\"Out2\",\"Out3\",\"Out1\"],\"side\":\"RIGHT\"},\"type\":\"ConnectorPlacement.EquallySpacedRectSide\",\"uuid\":\"cb1c6840-c5bf-4913-92c2-1c054d368f87\"},{\"content\":{\"side\":\"TOP\"},\"type\":\"ConnectorPlacement.EquallySpacedRectSide\",\"uuid\":\"3633cd87-b3f9-48c9-80b7-73d7f17aa7ad\"}]},\"type\":\"ConnectorPlacement.EquallySpacedConnector\",\"uuid\":\"2553d532-cb7a-499b-b98c-b91f81677a07\"}],\"packageUris\":[\"http://schema.mathworks.com/mf0/Connector/R2020b\"],\"version\":\"1.0\"}"
  CameraScheduler7 : Stateflow chart  TreatAsAtomicUnit=on
      settings: PortSchema="{\"entries\":[{\"content\":{\"sides\":[{\"content\":{\"connectorIds\":[\"In1\"]},\"type\":\"ConnectorPlacement.EquallySpacedRectSide\",\"uuid\":\"335362b2-4c4f-40e6-baf0-d287f6971824\"},{\"content\":{\"connectorIds\":[\"Out2\",\"Out1\"],\"side\":\"RIGHT\"},\"type\":\"ConnectorPlacement.EquallySpacedRectSide\",\"uuid\":\"7ee54d08-aa3e-4d6f-8253-6f749626479a\"},{\"content\":{\"side\":\"TOP\"},\"type\":\"ConnectorPlacement.EquallySpacedRectSide\",\"uuid\":\"7bf47310-47f4-4483-b0d1-b8a087b66b77\"}]},\"type\":\"ConnectorPlacement.EquallySpacedConnector\",\"uuid\":\"fb61df21-9632-41f0-9cfa-ce5060944b6c\"}],\"packageUris\":[\"http://schema.mathworks.com/mf0/Connector/R2020b\"],\"version\":\"1.0\"}"
  CameraScheduler8 : Stateflow chart  TreatAsAtomicUnit=on
      settings: PortSchema="{\"entries\":[{\"content\":{\"sides\":[{\"content\":{\"connectorIds\":[\"In1\"]},\"type\":\"ConnectorPlacement.EquallySpacedRectSide\",\"uuid\":\"228150a7-62a2-46d0-a1ac-a8e868d835b5\"},{\"content\":{\"connectorIds\":[\"Out2\",\"Out1\"],\"side\":\"RIGHT\"},\"type\":\"ConnectorPlacement.EquallySpacedRectSide\",\"uuid\":\"cb1c6840-c5bf-4913-92c2-1c054d368f87\"},{\"content\":{\"side\":\"TOP\"},\"type\":\"ConnectorPlacement.EquallySpacedRectSide\",\"uuid\":\"3633cd87-b3f9-48c9-80b7-73d7f17aa7ad\"}]},\"type\":\"ConnectorPlacement.EquallySpacedConnector\",\"uuid\":\"2553d532-cb7a-499b-b98c-b91f81677a07\"}],\"packageUris\":[\"http://schema.mathworks.com/mf0/Connector/R2020b\"],\"version\":\"1.0\"}"
  CameraScheduler9 : Stateflow chart  TreatAsAtomicUnit=on
      settings: PortSchema="{\"entries\":[{\"content\":{\"sides\":[{\"content\":{\"connectorIds\":[\"In1\"]},\"type\":\"ConnectorPlacement.EquallySpacedRectSide\",\"uuid\":\"335362b2-4c4f-40e6-baf0-d287f6971824\"},{\"content\":{\"connectorIds\":[\"Out2\",\"Out1\"],\"side\":\"RIGHT\"},\"type\":\"ConnectorPlacement.EquallySpacedRectSide\",\"uuid\":\"7ee54d08-aa3e-4d6f-8253-6f749626479a\"},{\"content\":{\"side\":\"TOP\"},\"type\":\"ConnectorPlacement.EquallySpacedRectSide\",\"uuid\":\"7bf47310-47f4-4483-b0d1-b8a087b66b77\"}]},\"type\":\"ConnectorPlacement.EquallySpacedConnector\",\"uuid\":\"fb61df21-9632-41f0-9cfa-ce5060944b6c\"}],\"packageUris\":[\"http://schema.mathworks.com/mf0/Connector/R2020b\"],\"version\":\"1.0\"}"
  Edge : Stateflow chart  TreatAsAtomicUnit=on
  From Workspace : FromWorkspace  VariableName=arrive_time  OutDataTypeStr=double  SampleTime=-1  Interpolate=off  ZeroCross=off  OutputAfterFinalValue=Holding final value
  From Workspace1 : FromWorkspace  VariableName=visibility_time  OutDataTypeStr=double  SampleTime=-1  Interpolate=off  ZeroCross=off  OutputAfterFinalValue=Holding final value
  From Workspace10 : FromWorkspace  VariableName=timer_array_3
  From Workspace11 : FromWorkspace  VariableName=blurryness_array_4
  From Workspace12 : FromWorkspace  VariableName=networkloss_array_4
  From Workspace13 : FromWorkspace  VariableName=timer_array_4
  From Workspace14 : FromWorkspace  VariableName=timer_array_7
  From Workspace15 : FromWorkspace  VariableName=blurryness_array_8
  From Workspace16 : FromWorkspace  VariableName=networkloss_array_8
  From Workspace17 : FromWorkspace  VariableName=timer_array_8
  From Workspace18 : FromWorkspace  VariableName=blurryness_array_5
  From Workspace19 : FromWorkspace  VariableName=networkloss_array_5
  From Workspace2 : FromWorkspace  VariableName=blurryness_array_1
  From Workspace20 : FromWorkspace  VariableName=timer_array_5
  From Workspace21 : FromWorkspace  VariableName=blurryness_array_6
  From Workspace22 : FromWorkspace  VariableName=networkloss_array_6
  From Workspace23 : FromWorkspace  VariableName=timer_array_6
  From Workspace24 : FromWorkspace  VariableName=blurryness_array_7
  From Workspace25 : FromWorkspace  VariableName=networkloss_array_7
  From Workspace26 : FromWorkspace  VariableName=timer_array_11
  From Workspace27 : FromWorkspace  VariableName=blurryness_array_12
  From Workspace28 : FromWorkspace  VariableName=networkloss_array_12
  From Workspace29 : FromWorkspace  VariableName=timer_array_12
  From Workspace3 : FromWorkspace  VariableName=networkloss_array_1
  From Workspace30 : FromWorkspace  VariableName=timer_array_15
  From Workspace31 : FromWorkspace  VariableName=blurryness_array_16
  From Workspace32 : FromWorkspace  VariableName=networkloss_array_16
  From Workspace33 : FromWorkspace  VariableName=timer_array_16
  From Workspace34 : FromWorkspace  VariableName=blurryness_array_13
  From Workspace35 : FromWorkspace  VariableName=networkloss_array_13
  From Workspace36 : FromWorkspace  VariableName=blurryness_array_9
  From Workspace37 : FromWorkspace  VariableName=timer_array_13
  From Workspace38 : FromWorkspace  VariableName=blurryness_array_14
  From Workspace39 : FromWorkspace  VariableName=networkloss_array_14
  From Workspace4 : FromWorkspace  VariableName=timer_array_1
  From Workspace40 : FromWorkspace  VariableName=timer_array_14
  From Workspace41 : FromWorkspace  VariableName=blurryness_array_15
  From Workspace42 : FromWorkspace  VariableName=networkloss_array_15
  From Workspace43 : FromWorkspace  VariableName=networkloss_array_9
  From Workspace44 : FromWorkspace  VariableName=timer_array_9
  From Workspace45 : FromWorkspace  VariableName=blurryness_array_10
  From Workspace46 : FromWorkspace  VariableName=networkloss_array_10
  From Workspace47 : FromWorkspace  VariableName=timer_array_10
  From Workspace48 : FromWorkspace  VariableName=blurryness_array_11
  From Workspace49 : FromWorkspace  VariableName=networkloss_array_11
  From Workspace5 : FromWorkspace  VariableName=blurryness_array_2
  From Workspace6 : FromWorkspace  VariableName=networkloss_array_2
  From Workspace7 : FromWorkspace  VariableName=timer_array_2
  From Workspace8 : FromWorkspace  VariableName=blurryness_array_3
  From Workspace9 : FromWorkspace  VariableName=networkloss_array_3
  Scope{,1..6} (7 alike) : Scope
  To Workspace : ToWorkspace  VariableName=faults  SaveFormat=Timeseries  SampleTime=-1
  Traffic : Stateflow chart  TreatAsAtomicUnit=on
  wires:
  From Workspace/1 -> Traffic/1(arrive_time)
  From Workspace1/1 -> Traffic/2(visibility_time)
  From Workspace2/1 -> CameraDriver/3(blurryness)
  CameraControl/1(image_request) -> CameraDriver/1(image_request)
  From Workspace3/1 -> CameraControl/2(network_faults)
  From Workspace4/1 -> CameraScheduler/1(timer_array)
  CameraDriver/1(image) -> CameraControl/1(imageIn)
  Edge/1(faults) -> Scope/1, To Workspace/1
  CameraControl1/2(imageOut) -> Edge/3(image2)
  CameraDriver1/1(image) -> CameraControl1/1(imageIn)
  From Workspace7/1 -> CameraScheduler1/1(timer_array)
  From Workspace6/1 -> CameraControl1/2(network_faults)
  CameraControl1/1(image_request) -> CameraDriver1/1(image_request)
  From Workspace5/1 -> CameraDriver1/3(blurryness)
  CameraControl/2(imageOut) -> Edge/2(image1)
  CameraScheduler/1(schedule_driver) -> CameraDriver/4(schedule)
  CameraScheduler1/2(schedule_control) -> CameraControl1/3(schedule)
  CameraScheduler1/1(schedule_driver) -> CameraDriver1/4(schedule)
  CameraScheduler/2(schedule_control) -> CameraControl/3(schedule)
  Edge/2(wait_time) -> Scope1/1
  CameraScheduler/3(i) -> Scope3/1
  CameraScheduler2/3(i) -> Scope4/1
  CameraScheduler2/2(schedule_control) -> CameraControl2/3(schedule)
  CameraScheduler3/1(schedule_driver) -> CameraDriver3/4(schedule)
  CameraScheduler3/2(schedule_control) -> CameraControl3/3(schedule)
  CameraScheduler2/1(schedule_driver) -> CameraDriver2/4(schedule)
  From Workspace11/1 -> CameraDriver3/3(blurryness)
  CameraControl3/1(image_request) -> CameraDriver3/1(image_request)
  From Workspace12/1 -> CameraControl3/2(network_faults)
  From Workspace13/1 -> CameraScheduler3/1(timer_array)
  CameraDriver3/1(image) -> CameraControl3/1(imageIn)
  CameraControl3/2(imageOut) -> Edge/5(image4)
  CameraDriver2/1(image) -> CameraControl2/1(imageIn)
  From Workspace10/1 -> CameraScheduler2/1(timer_array)
  From Workspace9/1 -> CameraControl2/2(network_faults)
  CameraControl2/1(image_request) -> CameraDriver2/1(image_request)
  From Workspace8/1 -> CameraDriver2/3(blurryness)
  CameraControl2/2(imageOut) -> Edge/4(image3)
  From Workspace24/1 -> CameraDriver6/3(blurryness)
  CameraControl6/1(image_request) -> CameraDriver6/1(image_request)
  From Workspace25/1 -> CameraControl6/2(network_faults)
  From Workspace14/1 -> CameraScheduler6/1(timer_array)
  CameraDriver6/1(image) -> CameraControl6/1(imageIn)
  CameraDriver7/1(image) -> CameraControl7/1(imageIn)
  From Workspace17/1 -> CameraScheduler7/1(timer_array)
  From Workspace16/1 -> CameraControl7/2(network_faults)
  CameraControl7/1(image_request) -> CameraDriver7/1(image_request)
  From Workspace15/1 -> CameraDriver7/3(blurryness)
  CameraScheduler6/1(schedule_driver) -> CameraDriver6/4(schedule)
  CameraScheduler7/2(schedule_control) -> CameraControl7/3(schedule)
  CameraScheduler7/1(schedule_driver) -> CameraDriver7/4(schedule)
  CameraScheduler6/2(schedule_control) -> CameraControl6/3(schedule)
  CameraScheduler6/3(i) -> Scope6/1
  CameraScheduler4/3(i) -> Scope5/1
  CameraScheduler4/2(schedule_control) -> CameraControl4/3(schedule)
  CameraScheduler5/1(schedule_driver) -> CameraDriver5/4(schedule)
  CameraScheduler5/2(schedule_control) -> CameraControl5/3(schedule)
  CameraScheduler4/1(schedule_driver) -> CameraDriver4/4(schedule)
  From Workspace21/1 -> CameraDriver5/3(blurryness)
  CameraControl5/1(image_request) -> CameraDriver5/1(image_request)
  From Workspace22/1 -> CameraControl5/2(network_faults)
  From Workspace23/1 -> CameraScheduler5/1(timer_array)
  CameraDriver5/1(image) -> CameraControl5/1(imageIn)
  CameraDriver4/1(image) -> CameraControl4/1(imageIn)
  From Workspace20/1 -> CameraScheduler4/1(timer_array)
  From Workspace19/1 -> CameraControl4/2(network_faults)
  CameraControl4/1(image_request) -> CameraDriver4/1(image_request)
  From Workspace18/1 -> CameraDriver4/3(blurryness)
  CameraControl4/2(imageOut) -> Edge/6(image5)
  CameraControl5/2(imageOut) -> Edge/7(image6)
  CameraControl6/2(imageOut) -> Edge/8(image7)
  CameraControl7/2(imageOut) -> Edge/9(image8)
  From Workspace34/1 -> CameraDriver12/3(blurryness)
  CameraControl12/1(image_request) -> CameraDriver12/1(image_request)
  From Workspace35/1 -> CameraControl12/2(network_faults)
  From Workspace37/1 -> CameraScheduler12/1(timer_array)
  CameraDriver12/1(image) -> CameraControl12/1(imageIn)
  CameraDriver13/1(image) -> CameraControl13/1(imageIn)
  From Workspace40/1 -> CameraScheduler13/1(timer_array)
  From Workspace39/1 -> CameraControl13/2(network_faults)
  CameraControl13/1(image_request) -> CameraDriver13/1(image_request)
  From Workspace38/1 -> CameraDriver13/3(blurryness)
  CameraScheduler12/1(schedule_driver) -> CameraDriver12/4(schedule)
  CameraScheduler13/2(schedule_control) -> CameraControl13/3(schedule)
  CameraScheduler13/1(schedule_driver) -> CameraDriver13/4(schedule)
  CameraScheduler12/2(schedule_control) -> CameraControl12/3(schedule)
  CameraScheduler14/2(schedule_control) -> CameraControl14/3(schedule)
  CameraScheduler15/1(schedule_driver) -> CameraDriver15/4(schedule)
  CameraScheduler15/2(schedule_control) -> CameraControl15/3(schedule)
  CameraScheduler14/1(schedule_driver) -> CameraDriver14/4(schedule)
  From Workspace31/1 -> CameraDriver15/3(blurryness)
  Traffic/1(traffic_state) -> CameraDriver/2(traffic_state), CameraDriver2/2(traffic_state), CameraDriver3/2(traffic_state), CameraDriver7/2(traffic_state), CameraDriver9/2(traffic_state), CameraDriver13/2(traffic_state), CameraDriver14/2(traffic_state), CameraDriver15/2(traffic_state), CameraDriver12/2(traffic_state), CameraDriver11/2(traffic_state), CameraDriver10/2(traffic_state), CameraDriver8/2(traffic_state), CameraDriver6/2(traffic_state), CameraDriver5/2(traffic_state), CameraDriver4/2(traffic_state), CameraDriver1/2(traffic_state), Scope2/1, Edge/1(traffic_state)
  CameraControl15/1(image_request) -> CameraDriver15/1(image_request)
  From Workspace32/1 -> CameraControl15/2(network_faults)
  From Workspace33/1 -> CameraScheduler15/1(timer_array)
  CameraDriver15/1(image) -> CameraControl15/1(imageIn)
  CameraDriver14/1(image) -> CameraControl14/1(imageIn)
  From Workspace30/1 -> CameraScheduler14/1(timer_array)
  From Workspace42/1 -> CameraControl14/2(network_faults)
  CameraControl14/1(image_request) -> CameraDriver14/1(image_request)
  From Workspace41/1 -> CameraDriver14/3(blurryness)
  From Workspace48/1 -> CameraDriver10/3(blurryness)
  CameraControl10/1(image_request) -> CameraDriver10/1(image_request)
  From Workspace49/1 -> CameraControl10/2(network_faults)
  From Workspace26/1 -> CameraScheduler10/1(timer_array)
  CameraDriver10/1(image) -> CameraControl10/1(imageIn)
  CameraDriver11/1(image) -> CameraControl11/1(imageIn)
  From Workspace29/1 -> CameraScheduler11/1(timer_array)
  From Workspace28/1 -> CameraControl11/2(network_faults)
  CameraControl11/1(image_request) -> CameraDriver11/1(image_request)
  From Workspace27/1 -> CameraDriver11/3(blurryness)
  CameraScheduler10/1(schedule_driver) -> CameraDriver10/4(schedule)
  CameraScheduler11/2(schedule_control) -> CameraControl11/3(schedule)
  CameraScheduler11/1(schedule_driver) -> CameraDriver11/4(schedule)
  CameraScheduler10/2(schedule_control) -> CameraControl10/3(schedule)
  CameraScheduler8/2(schedule_control) -> CameraControl8/3(schedule)
  CameraScheduler9/1(schedule_driver) -> CameraDriver9/4(schedule)
  CameraScheduler9/2(schedule_control) -> CameraControl9/3(schedule)
  CameraScheduler8/1(schedule_driver) -> CameraDriver8/4(schedule)
  From Workspace45/1 -> CameraDriver9/3(blurryness)
  CameraControl9/1(image_request) -> CameraDriver9/1(image_request)
  From Workspace46/1 -> CameraControl9/2(network_faults)
  From Workspace47/1 -> CameraScheduler9/1(timer_array)
  CameraDriver9/1(image) -> CameraControl9/1(imageIn)
  CameraDriver8/1(image) -> CameraControl8/1(imageIn)
  From Workspace44/1 -> CameraScheduler8/1(timer_array)
  From Workspace43/1 -> CameraControl8/2(network_faults)
  CameraControl8/1(image_request) -> CameraDriver8/1(image_request)
  From Workspace36/1 -> CameraDriver8/3(blurryness)
  CameraControl8/2(imageOut) -> Edge/10(image9)
  CameraControl9/2(imageOut) -> Edge/11(image10)
  CameraControl10/2(imageOut) -> Edge/12(image11)
  CameraControl11/2(imageOut) -> Edge/13(image12)
  CameraControl12/2(imageOut) -> Edge/14(image13)
  CameraControl13/2(imageOut) -> Edge/15(image14)
  CameraControl14/2(imageOut) -> Edge/16(image15)
  CameraControl15/2(imageOut) -> Edge/17(image16)
